simulink model "ON"  (R2025b)
settings: Solver=VariableStepAuto  StartTime=0.0  StopTime=165.5984  FixedStep=0.5  RelTol=1e-3
InitFcn:
  | createRefStates;
  | mdlWks = get_param(gcs,'ModelWorkspace');
  | a = getVariable(mdlWks,'a');
  | b = getVariable(mdlWks,'b');
  | c = getVariable(mdlWks,'c');
StopFcn:
  | fTraj = findobj("Tag","asbAUVTrajectory");
  | 
  | if isempty(fTraj)
  |    fTraj = figure("Tag","asbAUVTrajectory");
  |    axes(fTraj);
  | end
  | 
  | axTraj= gca(fTraj);
  | 
  | if exist('PositionData', 'var')
  |     % plot the intermediate points in yellow
  | 
  |    if d.Data == 1
  |       plot3(axTraj,ref_positions_x,ref_positions_y,ref_positions_z,'y*')
  |       hold on
  |       plot3(axTraj,PositionData(1,1),PositionData(1,2),PositionData(1,3),'r*')
  |       plot3(axTraj,PositionData(:,1),PositionData(:,2),PositionData(:,3));
  |       plot3(axTraj,PositionData(end,1),PositionData(end,2),PositionData(end,3),'g*');
  |       view(axTraj, 3);
  |    else
  |       plot(axTraj,ref_positions_x,ref_positions_y,'y*')
  |       hold on
  |       plot(axTraj,PositionData(1,1),PositionData(1,2),'r*')
  |       plot(axTraj,PositionData(:,1),PositionData(:,2));
  |       plot(axTraj,PositionData(end,1),PositionData(end,2),'g*');
  |       view(axTraj, 2);
  |    end
  | 
  | 
  | 
  | if exist("imu_acc", "var")
  | skip = 1;
  | N  = size(imu_acc.Data,1);
  | dt = (20/N)*skip;
  | T = N*dt;
  | 
  | % disp(["N", num2str(N)]);
  | % disp(["total time", num2str(T)]);
  | 
  | acc_bias = [0.0002;-0.00015;0.0001];
  | 
  | %% State vector
  | % x = [x y z vx vy vz bax bay baz]
  | n = 9;
  | 
  | %% True initial state
  | % x_true = [0;0;0;1;0.5;0.2];
  | 
  | %% Initial estimate
  | x_est = [PositionData(1,:)'; zeros(n-3,1)];
  | 
  | %% Initial covariance
  | P = 0.1*eye(n)*1;
  | 
  | %% Process noise
  | Q = diag([0 0 0 0.01 0.01 0.01 1e-6 1e-6 1e-6]);
  | % Q = diag([0 0 0 0.0 0.0 0.0 0 0 0]);
  | 
  | %% IMU noise
  | imu_noise = 0.02;
  | ... (+134 lines)
model workspace (MAT data in the model file):
  a = 0
  b = 1
  c = 1
  d = 0
values from neighbouring files (symbols this model uses):
  current_field = Config.water_current_params.field    [asbAUVax.m]
  data = [ ref_positions_x,           ref_positions_y,           ref_positions_z ]    [createRefStates.m]    (also in createRefStates_2D.m)
  imu_acc = acc_true + true_acc_bias + imu_noise*randn(3,1)    [covariance_examples.m]
  sampleTime = 0.1    [createRefStates.m]    (also in createRefStates_2D.m = 0.01)
  water_current_params = []    [createRefStates.m]
undefined symbols (not defined in the file or in its folder): obstacle_params
libraries: asbAUVlib x26, slpidlib x12, dspfdesign x6, aerolibobsolete x1, aerolibasang x1, sharedutil x1, aerolibnav x1, SignalEditorBlockLib x1
(part 3 of 3)

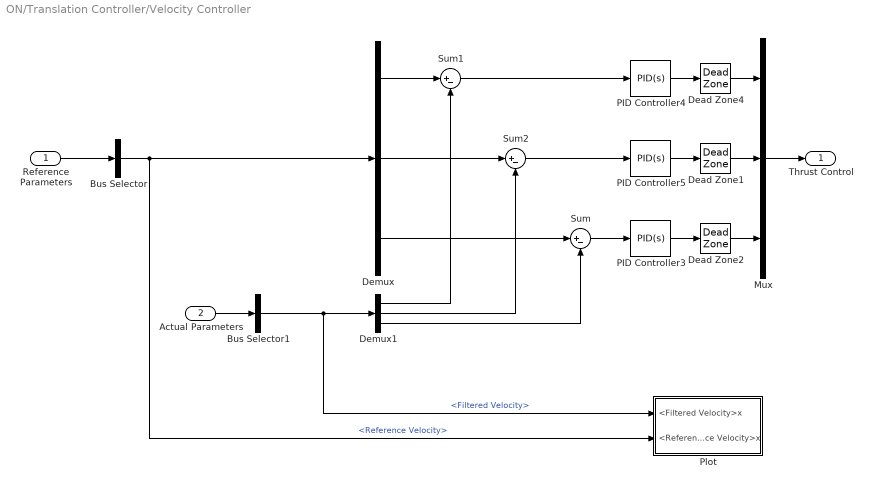
== system ON/Translation Controller/Velocity Controller ==
  Reference Parameters : Inport
  Actual Parameters : Inport  Port=2
  Bus Selector : BusSelector  OutputSignals=Reference Velocity
  Bus Selector1 : BusSelector  OutputSignals=Filtered Velocity
  Dead Zone1 : DeadZone  LowerValue=-0.05  UpperValue=+0.05
  Dead Zone2 : DeadZone  LowerValue=-0.05  UpperValue=+0.05
  Dead Zone4 : DeadZone  LowerValue=-0.05  UpperValue=+0.05
  Demux : Demux  Outputs=3
  Demux1 : Demux  Outputs=3
  Mux : Mux  Inputs=3
  PID Controller3 : slpidlib/PID Controller  Controller=PID  Form=Parallel  TimeDomain=Continuous-time  UseExternalTs=off  SampleTime=-1  IntegratorMethod=Forward Euler  FilterMethod=Forward Euler  ControllerParametersSource=internal  P=-0.61964554396314  I=-0.140214385843897  UseKiTs=off  D=0.00440045709674139  UseExternalDerivativeSource=off  N=140.813904178727  UseFilter=on  TunerSelectOption=Transfer Function Based (PID Tuner App)  InitialConditionSource=internal  InitialConditionForIntegrator=0  InitialConditionForFilter=0  DifferentiatorICPrevScaledInput=0  ExternalReset=none  TrackingMode=off  Kt=1  LimitOutput=off  SatLimitsSource=internal  UpperSaturationLimit=inf  LowerSaturationLimit=-inf  LinearizeAsGain=on  AntiWindupMode=none  Kb=1  LimitIntegrator=off  UpperIntegratorSaturationLimit=inf  LowerIntegratorSaturationLimit=-inf  POutMin=[]  POutMax=[]  IOutMin=[]  IOutMax=[]  DOutMin=[]  DOutMax=[]  NOutMin=[]  NOutMax=[]  SumOutMin=[]  SumOutMax=[]  SaturationOutMin=[]  SaturationOutMax=[]  PParamMin=[]  PParamMax=[]  IParamMin=[]  IParamMax=[]  DParamMin=[]  DParamMax=[]  NParamMin=[]  NParamMax=[]  KbParamMin=[]  KbParamMax=[]  KtParamMin=[]  KtParamMax=[]  KbOutMin=[]  KbOutMax=[]  KtOutMin=[]  KtOutMax=[]  IntegratorOutMin=[]  IntegratorOutMax=[]  FilterOutMin=[]  FilterOutMax=[]  SumI1OutMin=[]  SumI1OutMax=[]  SumI2OutMin=[]  SumI2OutMax=[]  SumI3OutMin=[]  SumI3OutMax=[]  SumI4OutMin=[]  SumI4OutMax=[]  SumDOutMin=[]  SumDOutMax=[]  DifferentiatorOutMin=[]  DifferentiatorOutMax=[]  FilterDiffOutCoefMin=[]  FilterDiffOutCoefMax=[]  ReciprocalOutMin=[]  ReciprocalOutMax=[]  SumDenOutMin=[]  SumDenOutMax=[]  SumNumOutMin=[]  SumNumOutMax=[]  DivideOutMin=[]  DivideOutMax=[]  UdiffTsProdOutMin=[]  UdiffTsProdOutMax=[]  NTsProdOutMin=[]  NTsProdOutMax=[]  UintegralTsProdOutMin=[]  UintegralTsProdOutMax=[]  UngainTsProdOutMin=[]  UngainTsProdOutMax=[]  ClampingZeroOutDataTypeStr=Inherit: Inherit via back propagation  ClampingZeroOutMin=[]  ClampingZeroOutMax=[]  FilterDenConstantOutDataTypeStr=Inherit: Inherit via back propagation  FilterDenConstantOutMin=[]  FilterDenConstantOutMax=[]  PCopyOutDataTypeStr=Inherit: Inherit via back propagation  PCopyOutMin=[]  PCopyOutMax=[]  NCopyOutDataTypeStr=Inherit: Inherit via back propagation  NCopyOutMin=[]  NCopyOutMax=[]  IntegratorContinuousStateAttributes=''  IntegratorStateMustResolveToSignalObject=off  IntegratorRTWStateStorageClass=Auto  FilterContinuousStateAttributes=''  FilterStateMustResolveToSignalObject=off  FilterRTWStateStorageClass=Auto  ParallelPVariant=InternalParameters  IdealPVariant=Disabled  IVariant=InternalParameters  DVariant=InternalParameters  IntegratorVariant=Continuous  SatVariant=Disabled  AWVariant=Passthrough  PCopyVariant=Disabled  TRVariant=Disabled  FdbkBlocksVariant=Forward  IdealPFdbkVariant=Disabled  SatFdbkVariant=Disabled  DerivativeFilterVariant=ContFilter  NVariant=InternalParameters  NCopyVariant=Disabled  FilterICVariant=InternalICsFilter  IntegratorICVariant=InternalICs  ExternalResetVariant=Disabled  TRSumVariant=Passthrough  SumFdbkVariant=Disabled  SumVariant=Sum_PID  TsampFilterVariant=InternalTs  TsampNgainVariant=Passthrough  TsampIntegralVariant=Disabled_SignalSpec  ExternalSaturationOutDataTypeStr=Inherit: Same as second input  DerivativeSourceVariant=ErrorSignal  PreIntVariant=InternalPreInt
  PID Controller4 : slpidlib/PID Controller  Controller=PID  Form=Parallel  TimeDomain=Continuous-time  UseExternalTs=off  SampleTime=-1  IntegratorMethod=Forward Euler  FilterMethod=Forward Euler  ControllerParametersSource=internal  P=0.262050505979025  I=0.0518732197045156  UseKiTs=off  D=-0.0235509594288088  UseExternalDerivativeSource=off  N=11.1269567072699  UseFilter=on  TunerSelectOption=Transfer Function Based (PID Tuner App)  InitialConditionSource=internal  InitialConditionForIntegrator=0  InitialConditionForFilter=0  DifferentiatorICPrevScaledInput=0  ExternalReset=none  TrackingMode=off  Kt=1  LimitOutput=off  SatLimitsSource=internal  UpperSaturationLimit=inf  LowerSaturationLimit=-inf  LinearizeAsGain=on  AntiWindupMode=none  Kb=1  LimitIntegrator=off  UpperIntegratorSaturationLimit=inf  LowerIntegratorSaturationLimit=-inf  POutMin=[]  POutMax=[]  IOutMin=[]  IOutMax=[]  DOutMin=[]  DOutMax=[]  NOutMin=[]  NOutMax=[]  SumOutMin=[]  SumOutMax=[]  SaturationOutMin=[]  SaturationOutMax=[]  PParamMin=[]  PParamMax=[]  IParamMin=[]  IParamMax=[]  DParamMin=[]  DParamMax=[]  NParamMin=[]  NParamMax=[]  KbParamMin=[]  KbParamMax=[]  KtParamMin=[]  KtParamMax=[]  KbOutMin=[]  KbOutMax=[]  KtOutMin=[]  KtOutMax=[]  IntegratorOutMin=[]  IntegratorOutMax=[]  FilterOutMin=[]  FilterOutMax=[]  SumI1OutMin=[]  SumI1OutMax=[]  SumI2OutMin=[]  SumI2OutMax=[]  SumI3OutMin=[]  SumI3OutMax=[]  SumI4OutMin=[]  SumI4OutMax=[]  SumDOutMin=[]  SumDOutMax=[]  DifferentiatorOutMin=[]  DifferentiatorOutMax=[]  FilterDiffOutCoefMin=[]  FilterDiffOutCoefMax=[]  ReciprocalOutMin=[]  ReciprocalOutMax=[]  SumDenOutMin=[]  SumDenOutMax=[]  SumNumOutMin=[]  SumNumOutMax=[]  DivideOutMin=[]  DivideOutMax=[]  UdiffTsProdOutMin=[]  UdiffTsProdOutMax=[]  NTsProdOutMin=[]  NTsProdOutMax=[]  UintegralTsProdOutMin=[]  UintegralTsProdOutMax=[]  UngainTsProdOutMin=[]  UngainTsProdOutMax=[]  ClampingZeroOutDataTypeStr=Inherit: Inherit via back propagation  ClampingZeroOutMin=[]  ClampingZeroOutMax=[]  FilterDenConstantOutDataTypeStr=Inherit: Inherit via back propagation  FilterDenConstantOutMin=[]  FilterDenConstantOutMax=[]  PCopyOutDataTypeStr=Inherit: Inherit via back propagation  PCopyOutMin=[]  PCopyOutMax=[]  NCopyOutDataTypeStr=Inherit: Inherit via back propagation  NCopyOutMin=[]  NCopyOutMax=[]  IntegratorContinuousStateAttributes=''  IntegratorStateMustResolveToSignalObject=off  IntegratorRTWStateStorageClass=Auto  FilterContinuousStateAttributes=''  FilterStateMustResolveToSignalObject=off  FilterRTWStateStorageClass=Auto  ParallelPVariant=InternalParameters  IdealPVariant=Disabled  IVariant=InternalParameters  DVariant=InternalParameters  IntegratorVariant=Continuous  SatVariant=Disabled  AWVariant=Passthrough  PCopyVariant=Disabled  TRVariant=Disabled  FdbkBlocksVariant=Forward  IdealPFdbkVariant=Disabled  SatFdbkVariant=Disabled  DerivativeFilterVariant=ContFilter  NVariant=InternalParameters  NCopyVariant=Disabled  FilterICVariant=InternalICsFilter  IntegratorICVariant=InternalICs  ExternalResetVariant=Disabled  TRSumVariant=Passthrough  SumFdbkVariant=Disabled  SumVariant=Sum_PID  TsampFilterVariant=InternalTs  TsampNgainVariant=Passthrough  TsampIntegralVariant=Disabled_SignalSpec  ExternalSaturationOutDataTypeStr=Inherit: Same as second input  DerivativeSourceVariant=ErrorSignal  PreIntVariant=InternalPreInt
  PID Controller5 : slpidlib/PID Controller  Controller=PID  Form=Parallel  TimeDomain=Continuous-time  UseExternalTs=off  SampleTime=-1  IntegratorMethod=Forward Euler  FilterMethod=Forward Euler  ControllerParametersSource=internal  P=1.14371295451496  I=0.548529610159355  UseKiTs=off  D=-0.00383210771245667  UseExternalDerivativeSource=off  N=298.455325458939  UseFilter=on  TunerSelectOption=Transfer Function Based (PID Tuner App)  InitialConditionSource=internal  InitialConditionForIntegrator=0  InitialConditionForFilter=0  DifferentiatorICPrevScaledInput=0  ExternalReset=none  TrackingMode=off  Kt=1  LimitOutput=off  SatLimitsSource=internal  UpperSaturationLimit=inf  LowerSaturationLimit=-inf  LinearizeAsGain=on  AntiWindupMode=none  Kb=1  LimitIntegrator=off  UpperIntegratorSaturationLimit=inf  LowerIntegratorSaturationLimit=-inf  POutMin=[]  POutMax=[]  IOutMin=[]  IOutMax=[]  DOutMin=[]  DOutMax=[]  NOutMin=[]  NOutMax=[]  SumOutMin=[]  SumOutMax=[]  SaturationOutMin=[]  SaturationOutMax=[]  PParamMin=[]  PParamMax=[]  IParamMin=[]  IParamMax=[]  DParamMin=[]  DParamMax=[]  NParamMin=[]  NParamMax=[]  KbParamMin=[]  KbParamMax=[]  KtParamMin=[]  KtParamMax=[]  KbOutMin=[]  KbOutMax=[]  KtOutMin=[]  KtOutMax=[]  IntegratorOutMin=[]  IntegratorOutMax=[]  FilterOutMin=[]  FilterOutMax=[]  SumI1OutMin=[]  SumI1OutMax=[]  SumI2OutMin=[]  SumI2OutMax=[]  SumI3OutMin=[]  SumI3OutMax=[]  SumI4OutMin=[]  SumI4OutMax=[]  SumDOutMin=[]  SumDOutMax=[]  DifferentiatorOutMin=[]  DifferentiatorOutMax=[]  FilterDiffOutCoefMin=[]  FilterDiffOutCoefMax=[]  ReciprocalOutMin=[]  ReciprocalOutMax=[]  SumDenOutMin=[]  SumDenOutMax=[]  SumNumOutMin=[]  SumNumOutMax=[]  DivideOutMin=[]  DivideOutMax=[]  UdiffTsProdOutMin=[]  UdiffTsProdOutMax=[]  NTsProdOutMin=[]  NTsProdOutMax=[]  UintegralTsProdOutMin=[]  UintegralTsProdOutMax=[]  UngainTsProdOutMin=[]  UngainTsProdOutMax=[]  ClampingZeroOutDataTypeStr=Inherit: Inherit via back propagation  ClampingZeroOutMin=[]  ClampingZeroOutMax=[]  FilterDenConstantOutDataTypeStr=Inherit: Inherit via back propagation  FilterDenConstantOutMin=[]  FilterDenConstantOutMax=[]  PCopyOutDataTypeStr=Inherit: Inherit via back propagation  PCopyOutMin=[]  PCopyOutMax=[]  NCopyOutDataTypeStr=Inherit: Inherit via back propagation  NCopyOutMin=[]  NCopyOutMax=[]  IntegratorContinuousStateAttributes=''  IntegratorStateMustResolveToSignalObject=off  IntegratorRTWStateStorageClass=Auto  FilterContinuousStateAttributes=''  FilterStateMustResolveToSignalObject=off  FilterRTWStateStorageClass=Auto  ParallelPVariant=InternalParameters  IdealPVariant=Disabled  IVariant=InternalParameters  DVariant=InternalParameters  IntegratorVariant=Continuous  SatVariant=Disabled  AWVariant=Passthrough  PCopyVariant=Disabled  TRVariant=Disabled  FdbkBlocksVariant=Forward  IdealPFdbkVariant=Disabled  SatFdbkVariant=Disabled  DerivativeFilterVariant=ContFilter  NVariant=InternalParameters  NCopyVariant=Disabled  FilterICVariant=InternalICsFilter  IntegratorICVariant=InternalICs  ExternalResetVariant=Disabled  TRSumVariant=Passthrough  SumFdbkVariant=Disabled  SumVariant=Sum_PID  TsampFilterVariant=InternalTs  TsampNgainVariant=Passthrough  TsampIntegralVariant=Disabled_SignalSpec  ExternalSaturationOutDataTypeStr=Inherit: Same as second input  DerivativeSourceVariant=ErrorSignal  PreIntVariant=InternalPreInt
  Plot : Subsystem  AncestorBlock=asbAUVlib/Plot
  Sum : Sum  Inputs=|+-
  Sum1 : Sum  Inputs=|+-
  Sum2 : Sum  Inputs=|+-
  Thrust Control : Outport  VectorParamsAs1DForOutWhenUnconnected=off
  wires:
  Demux1/3 -> Sum/2
  PID Controller3/1 -> Dead Zone2/1
  Demux/3 -> Sum/1
  PID Controller4/1 -> Dead Zone4/1
  PID Controller5/1 -> Dead Zone1/1
  Demux/2 -> Sum2/1
  Dead Zone2/1 -> Mux/3
  Dead Zone1/1 -> Mux/2
  Demux/1 -> Sum1/1
  Demux1/1 -> Sum1/2
  Demux1/2 -> Sum2/2
  Dead Zone4/1 -> Mux/1
  Mux/1 -> Thrust Control/1
  Sum1/1 -> PID Controller4/1
  Sum2/1 -> PID Controller5/1
  Sum/1 -> PID Controller3/1
  Bus Selector/1 -> Plot/2(<Reference Velocity>x), Demux/1  "<Reference Velocity>"
  Reference Parameters/1 -> Bus Selector/1
  Bus Selector1/1 -> Plot/1(<Filtered Velocity>x), Demux1/1  "<Filtered Velocity>"
  Actual Parameters/1 -> Bus Selector1/1

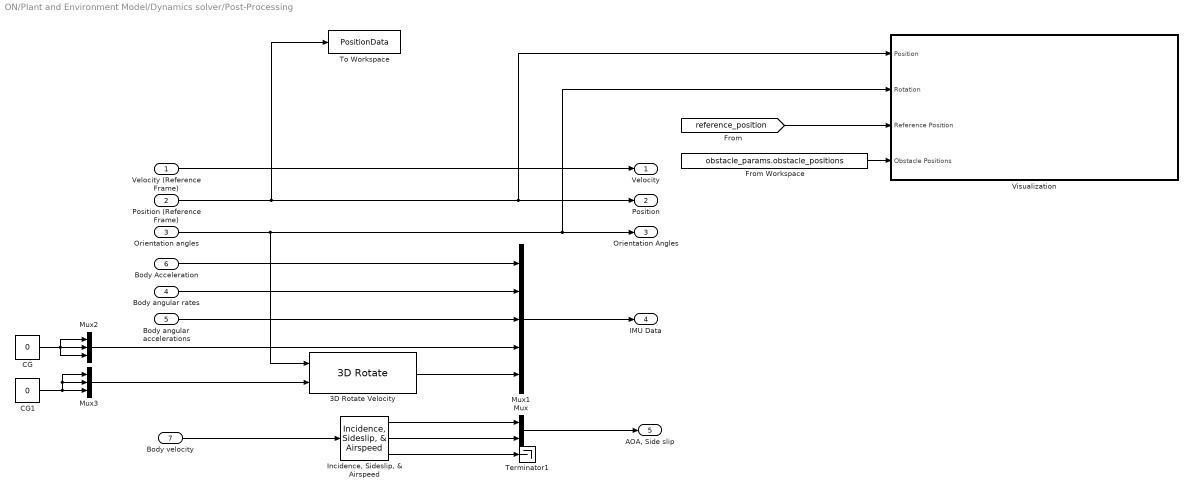
== system ON/Plant and Environment Model/Dynamics solver/Post-Processing ==
  Velocity (Reference Frame) : Inport
  Position (Reference Frame) : Inport  Port=2
  Orientation angles : Inport  Port=3
  Body angular rates : Inport  Port=4
  Body angular accelerations : Inport  Port=5
  Body Acceleration : Inport  Port=6
  Body velocity : Inport  Port=7
  3D Rotate Velocity : asbAUVlib/3D Rotate   SystemSampleTime=-1  VariantActivationTime=update diagram  EmptyChoice=off  PassThrough=off  PassThroughVariantControl=(default)  EmptyChoiceVariantControl=(default)  AllowFlexibleInterface=on  Latency=0  AutoFrameSizeCalculation=off
  CG : Constant  Value=0
  CG1 : Constant  Value=0
  From Workspace : FromWorkspace  VariableName=obstacle_params.obstacle_positions
  "Incidence, Sideslip, & Airspeed" : aerolibasang/Incidence, Sideslip, & Airspeed
  Mux : Mux  Inputs=2
  Mux1 : Mux  Inputs=5
  Mux2 : Mux  Inputs=3
  Mux3 : Mux  Inputs=3
  Terminator1 : Terminator
  To Workspace : ToWorkspace  VariableName=PositionData  SampleTime=-1
  Visualization : Subsystem  mask(6DoF_Animation){u2=sampleTime*10, u8=on, u9=d, u10=water_current_params, u11=obstacle_params}
      mask prompts: u2 "aeroblks:aeroblkanim6dof:block6DoF_AnimationParamTimeintervalbetweenupdates"; u8 "aeroblks:aeroblkanim6dof:block6DoF_AnimationParamEnableanimation"; u9 "2D or 3D plotting"; u10 "Water Current Parameters"; u11 "Obstacle Parameters"
      mask help: aeroblks:aeroblkanim6dof:block6DoF_AnimationDesc
      mask init:
      | aeroicon('aeroblk');
      | Config.update = u2;
      | Config.Animenable = u8;
      | Config.Model = bdroot(gcb);
      | Config.dimension = u9;
      | Config.water_current_params = u10;
      | Config.obstacle_params = u11;
      mask Help: eval('asbhelp(''sixdof_animation'')');
      mask DialogControl DescGroupVar Prompt: Animation
      mask DialogControl DescTextVar Prompt: Show animation of body
      mask DialogControl u2 Prompt: Time interval between updates:
      mask DialogControl u8 Prompt: Enable animation
      mask Display:
      | port_label('input',1,'x_e','texmode','on');
      | port_label('input',2,'\phi \theta \psi','texmode','on');
  Velocity : Outport  VectorParamsAs1DForOutWhenUnconnected=off
  " Position" : Outport  Port=2  VectorParamsAs1DForOutWhenUnconnected=off
  Orientation Angles : Outport  Port=3  VectorParamsAs1DForOutWhenUnconnected=off
  IMU Data : Outport  Port=4  VectorParamsAs1DForOutWhenUnconnected=off
  "AOA, Side slip" : Outport  Port=5  VectorParamsAs1DForOutWhenUnconnected=off
  wires:
  Body angular accelerations/1 -> Mux1/3
  "Incidence, Sideslip, & Airspeed"/2 -> Mux/2
  Body velocity/1 -> "Incidence, Sideslip, & Airspeed"/1
  "Incidence, Sideslip, & Airspeed"/1 -> Mux/1
  Body angular rates/1 -> Mux1/2
  CG/1 -> Mux2/2, Mux2/1, Mux2/3
  3D Rotate Velocity/1 -> Mux1/5
  Mux2/1 -> Mux1/4
  Mux/1 -> "AOA, Side slip"/1
  CG1/1 -> Mux3/2, Mux3/1, Mux3/3
  Mux3/1 -> 3D Rotate Velocity/2
  Body Acceleration/1 -> Mux1/1
  Velocity (Reference Frame)/1 -> Velocity/1
  Orientation angles/1 -> 3D Rotate Velocity/1, Visualization/2(Rotation), Orientation Angles/1
  Mux1/1 -> IMU Data/1
  "Incidence, Sideslip, & Airspeed"/3 -> Terminator1/1
  Position (Reference Frame)/1 -> " Position"/1, Visualization/1(Position), To Workspace/1
  [reference_position] -> Visualization/3(Reference Position)
  From Workspace/1 -> Visualization/4(Obstacle Positions)

== system ON/Plant and Environment Model/Environmental Forces & Moments/Hydrodynamic Forces ==
  "Submarine Velocity (Body Axis) " : Inport
  "AOA, Side Slip" : Inport  Port=2
  Hydrodynamic Forces - Accurate : Subsystem  VariantControl=b==1
  Hydrodynamic Forces - Basic : Subsystem  VariantControl=b==0
  "Force due to Lift, Drag" : Outport  VectorParamsAs1DForOutWhenUnconnected=off

== system ON/Plant and Environment Model/Environmental Forces & Moments/Hydrostatic Forces ==
  In1 : Inport
  Constant : Constant
  Environment Model : Subsystem  mask{ro=1000, V=0.01, M=10, a=0, b=0, c=0}
      mask prompts: ro "Density of Water"; V "Volume of Submarine"; M "Mass of Submarine"; a "X Distance between CG and CB"; b "Y Distance between CG and CB"; c "Z Distance between CG and CB"
      mask DialogControl DescTextVar Prompt: Enter the Submarine related Parameters
      mask DialogControl Container3 Prompt: Distance between CG and Center of Buoyancy
  Hydrostatic Force : Outport  VectorParamsAs1DForOutWhenUnconnected=off
  Hydrostatic Moment : Outport  Port=2  VectorParamsAs1DForOutWhenUnconnected=off
  wires:
  Constant/1 -> Environment Model/1("Fraction submerged ")
  Environment Model/2(Moment due to Weight and Buoyancy) -> Hydrostatic Moment/1
  Environment Model/1(Forces due to Weight and Buoyancy) -> Hydrostatic Force/1
  In1/1 -> Environment Model/2(Orientation Angles)

== system ON/Plant and Environment Model/Propulsion Forces & Moments/Force and moments due to Thrust ==
  Thrust Inputs : Inport
  "Thrust to Propulsion " : Subsystem
  Propulsion Force : Outport  VectorParamsAs1DForOutWhenUnconnected=off
  Propulsion Moment : Outport  Port=2  VectorParamsAs1DForOutWhenUnconnected=off
  wires:
  "Thrust to Propulsion "/2(Propulsion Moment) -> Propulsion Moment/1
  Thrust Inputs/1 -> "Thrust to Propulsion "/1(Thrust Inputs)
  "Thrust to Propulsion "/1(Propulsion Force) -> Propulsion Force/1

== system ON/Plant and Environment Model/Propulsion Forces & Moments/Input commands to Thrust ==
  Thrust Control Inputs : Inport
  Demux : Demux  Outputs=3
  Input Commands to PWM : Subsystem
  "PWM Signals to Thrust " : Subsystem
  Thrust values : Outport  VectorParamsAs1DForOutWhenUnconnected=off
  wires:
  Input Commands to PWM/1(Px1) -> "PWM Signals to Thrust "/1(PWM Signal Px1)
  Input Commands to PWM/3(Py1) -> "PWM Signals to Thrust "/3(PWM Signal Py1)
  Demux/1 -> Input Commands to PWM/1(X Thruster)  "X Thrust Input"
  Demux/3 -> Input Commands to PWM/3(Z Thruster)  "Z Thrust Input"
  Input Commands to PWM/4(Py2) -> "PWM Signals to Thrust "/4(PWM Signal Py2)
  Demux/2 -> Input Commands to PWM/2(Y Thruster)  "Y Thrust Input"
  Input Commands to PWM/2(Px2) -> "PWM Signals to Thrust "/2(PWM Signal Px2)
  Input Commands to PWM/5(Pz) -> "PWM Signals to Thrust "/5(PWM Signal Pz)
  "PWM Signals to Thrust "/1(Thrust (N)) -> Thrust values/1
  Thrust Control Inputs/1 -> Demux/1

== system ON/Sensor data and State Estimation/System With Noise/ Sensor (IMU) ==
  IMU Inputs : Inport
  Bus Creator : BusCreator  Inputs=2
  Bus Selector : BusSelector  OutputSignals=IMU Data
  Demux : Demux  Outputs=5
  Three-axis Inertial Measurement Unit : aerolibnav/Three-axis Inertial Measurement Unit  units=Metric (MKS)  imu=data(1,:)  i_Ts=0  dtype_a=on  w_a=190  z_a=0.707  a_sf_cc=[1 0 0; 0 1 0; 0 0 1]  a_bias=[0 0 0]  a_sat="[-inf  -inf  -inf  inf inf inf]"  dtype_g=on  w_g=190  z_g=0.707  g_sf_cc=[1 0 0; 0 1 0; 0 0 1]  g_bias=[0 0 0]  g_sens=[0 0 0]  g_sat="[-inf  -inf  -inf  inf inf inf]"  i_rand=on  i_seeds=[23093 23094 23095 23096 23097 23098]  i_pow=[0.00001 0.00001 0.00001 0.00001 0.00001 0.00001]
  IMU Measurements : Outport  VectorParamsAs1DForOutWhenUnconnected=off
  wires:
  Three-axis Inertial Measurement Unit/1 -> Bus Creator/1  "IMU Measured Acceleration"
  Demux/2 -> Three-axis Inertial Measurement Unit/2
  Demux/4 -> Three-axis Inertial Measurement Unit/4
  Demux/5 -> Three-axis Inertial Measurement Unit/5
  Demux/3 -> Three-axis Inertial Measurement Unit/3
  Demux/1 -> Three-axis Inertial Measurement Unit/1
  Three-axis Inertial Measurement Unit/2 -> Bus Creator/2  "IMU Measured Body Rates"
  IMU Inputs/1 -> Bus Selector/1
  Bus Selector/1 -> Demux/1  "<IMU Data>"
  Bus Creator/1 -> IMU Measurements/1

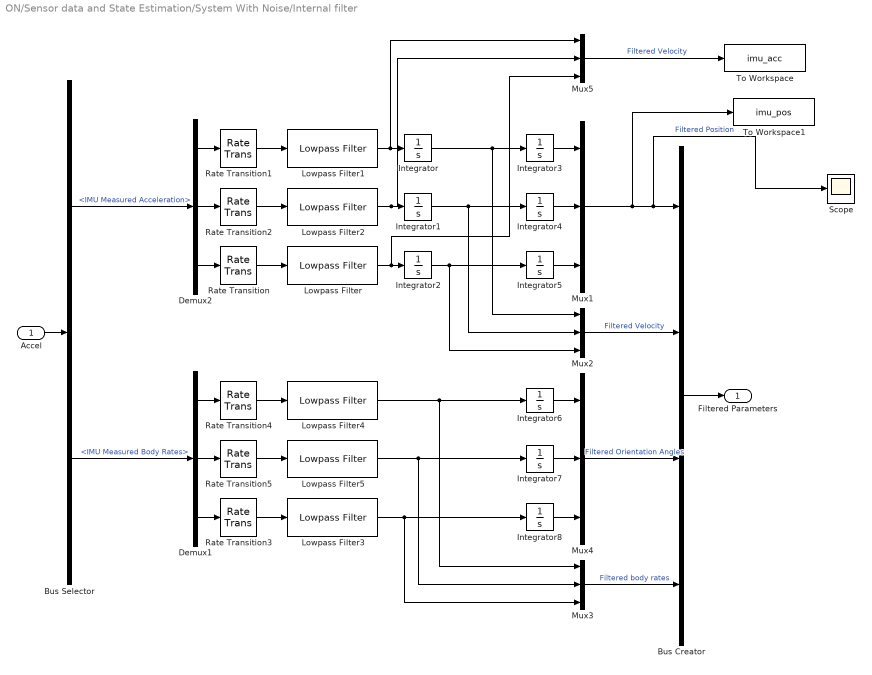
== system ON/Sensor data and State Estimation/System With Noise/Internal filter ==
  Accel : Inport
  Bus Creator : BusCreator  Inputs=4
  Bus Selector : BusSelector  OutputSignals=IMU Measured Acceleration,IMU Measured Body Rates
  Demux1 : Demux  Outputs=3
  Demux2 : Demux  Outputs=3
  Integrator{,1..2,6..8} (6 alike) : Integrator
  Integrator3 : Integrator  InitialCondition=data(1,1)
  Integrator4 : Integrator  InitialCondition=data(1,2)
  Integrator5 : Integrator  InitialCondition=data(1,3)
  Lowpass Filter{,1..5} (6 alike) : dspfdesign/Lowpass Filter  FilterType=FIR  DesignForMinimumOrder=on  FilterOrder=50  PassbandFrequency=1/100  StopbandFrequency=45  PassbandRipple=0.1  StopbandAttenuation=80  SampleRateMode=Specify on dialog  SampleRate=100  SimulateUsing=Interpreted execution  roundingMode=Floor  coeffsDataTypeStr=fixdt(1,16)
  Mux{1..5} (5 alike) : Mux  Inputs=3
  Rate Transition{,1..5} (6 alike) : RateTransition  OutPortSampleTime=0.01
  Scope : Scope
      settings: ActiveDisplayYMinimum=-560.24422155517175  ActiveDisplayYMaximum=62.268150319716625
  To Workspace : ToWorkspace  VariableName=imu_acc  SaveFormat=Timeseries  SampleTime=-1
  To Workspace1 : ToWorkspace  VariableName=imu_pos  SaveFormat=Timeseries  SampleTime=-1
  Filtered Parameters : Outport  VectorParamsAs1DForOutWhenUnconnected=off
  wires:
  Rate Transition5/1 -> Lowpass Filter5/1
  Rate Transition4/1 -> Lowpass Filter4/1
  Demux1/1 -> Rate Transition4/1
  Lowpass Filter3/1 -> Integrator8/1, Mux3/3
  Demux1/2 -> Rate Transition5/1
  Lowpass Filter5/1 -> Integrator7/1, Mux3/2
  Lowpass Filter4/1 -> Integrator6/1, Mux3/1
  Integrator6/1 -> Mux4/1
  Rate Transition3/1 -> Lowpass Filter3/1
  Integrator8/1 -> Mux4/3
  Demux1/3 -> Rate Transition3/1
  Integrator7/1 -> Mux4/2
  Accel/1 -> Bus Selector/1
  Bus Selector/1 -> Demux2/1  "<IMU Measured Acceleration>"
  Bus Selector/2 -> Demux1/1  "<IMU Measured Body Rates>"
  Mux4/1 -> Bus Creator/3  "Filtered Orientation Angles"
  Mux3/1 -> Bus Creator/4  "Filtered body rates"
  Bus Creator/1 -> Filtered Parameters/1
  Integrator2/1 -> Integrator5/1, Mux2/3
  Integrator/1 -> Integrator3/1, Mux2/1
  Mux2/1 -> Bus Creator/2  "Filtered Velocity"
  Mux1/1 -> To Workspace1/1, Scope/1, Bus Creator/1  "Filtered Position"
  Lowpass Filter/1 -> Mux5/3, Integrator2/1
  Demux2/2 -> Rate Transition2/1
  Rate Transition1/1 -> Lowpass Filter1/1
  Integrator4/1 -> Mux1/2
  Demux2/3 -> Rate Transition/1
  Lowpass Filter2/1 -> Mux5/2, Integrator1/1
  Lowpass Filter1/1 -> Mux5/1, Integrator/1
  Demux2/1 -> Rate Transition1/1
  Integrator5/1 -> Mux1/3
  Integrator1/1 -> Integrator4/1, Mux2/2
  Rate Transition/1 -> Lowpass Filter/1
  Integrator3/1 -> Mux1/1
  Rate Transition2/1 -> Lowpass Filter2/1
  Mux5/1 -> To Workspace/1  "Filtered Velocity"

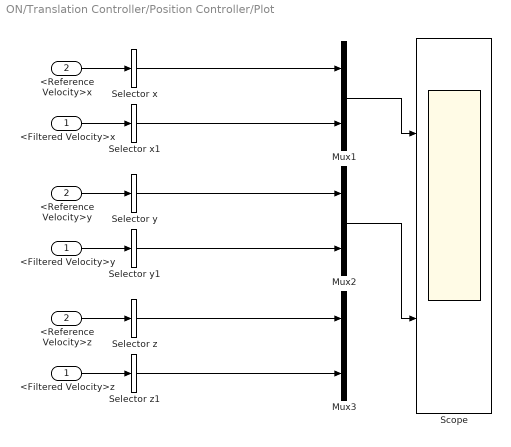
== system ON/Translation Controller/Position Controller/Plot ==
  <Filtered Velocity>x : Inport
  <Reference Velocity>x : Inport  Port=2
  <Filtered Velocity>y : InportShadow
  <Filtered Velocity>z : InportShadow
  <Reference Velocity>y : InportShadow  Port=2
  <Reference Velocity>z : InportShadow  Port=2
  Mux1 : Mux  Inputs=2
  Mux2 : Mux  Inputs=2
  Mux3 : Mux  Inputs=2
  Scope : Scope  NumInputPorts=2
      settings: ActiveDisplayYMinimum=-3.1120995154510725E+7  ActiveDisplayYMaximum=3.4601198502526991E+6
  Selector x : Selector  InputPortWidth=3  IndexOptions=Index vector (dialog)  Indices=1  OutputSizes=1
  Selector x1 : Selector  InputPortWidth=3  IndexOptions=Index vector (dialog)  Indices=1  OutputSizes=1
  Selector y : Selector  InputPortWidth=3  IndexOptions=Index vector (dialog)  Indices=2  OutputSizes=1
  Selector y1 : Selector  InputPortWidth=3  IndexOptions=Index vector (dialog)  Indices=2  OutputSizes=1
  Selector z : Selector  InputPortWidth=3  IndexOptions=Index vector (dialog)  Indices=2  OutputSizes=1
  Selector z1 : Selector  InputPortWidth=3  IndexOptions=Index vector (dialog)  Indices=2  OutputSizes=1
  wires:
  <Filtered Velocity>z/1 -> Selector z1/1
  <Filtered Velocity>y/1 -> Selector y1/1
  <Filtered Velocity>x/1 -> Selector x1/1
  <Reference Velocity>z/1 -> Selector z/1
  <Reference Velocity>y/1 -> Selector y/1
  <Reference Velocity>x/1 -> Selector x/1
  Selector z1/1 -> Mux3/2
  Selector x/1 -> Mux1/1
  Selector y/1 -> Mux2/1
  Mux1/1 -> Scope/1
  Mux2/1 -> Scope/2
  Selector z/1 -> Mux3/1
  Selector y1/1 -> Mux2/2
  Selector x1/1 -> Mux1/2

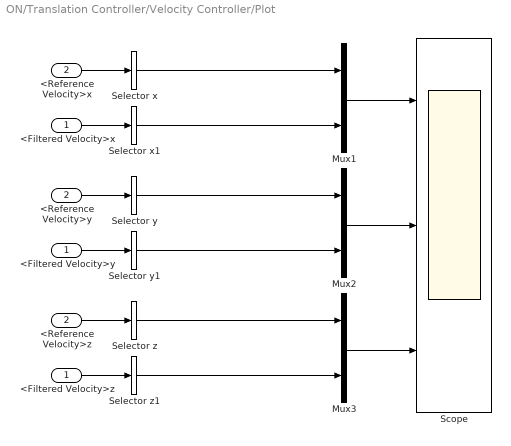
== system ON/Translation Controller/Velocity Controller/Plot ==
  <Filtered Velocity>x : Inport
  <Reference Velocity>x : Inport  Port=2
  <Filtered Velocity>y : InportShadow
  <Filtered Velocity>z : InportShadow
  <Reference Velocity>y : InportShadow  Port=2
  <Reference Velocity>z : InportShadow  Port=2
  Mux1 : Mux  Inputs=2
  Mux2 : Mux  Inputs=2
  Mux3 : Mux  Inputs=2
  Scope : Scope  NumInputPorts=3
      settings: ActiveDisplayYMinimum=-1  ActiveDisplayYMaximum=1
  Selector x : Selector  InputPortWidth=3  IndexOptions=Index vector (dialog)  Indices=1  OutputSizes=1
  Selector x1 : Selector  InputPortWidth=3  IndexOptions=Index vector (dialog)  Indices=1  OutputSizes=1
  Selector y : Selector  InputPortWidth=3  IndexOptions=Index vector (dialog)  Indices=2  OutputSizes=1
  Selector y1 : Selector  InputPortWidth=3  IndexOptions=Index vector (dialog)  Indices=2  OutputSizes=1
  Selector z : Selector  InputPortWidth=3  IndexOptions=Index vector (dialog)  Indices=2  OutputSizes=1
  Selector z1 : Selector  InputPortWidth=3  IndexOptions=Index vector (dialog)  Indices=2  OutputSizes=1
  wires:
  <Filtered Velocity>z/1 -> Selector z1/1
  <Filtered Velocity>y/1 -> Selector y1/1
  <Filtered Velocity>x/1 -> Selector x1/1
  <Reference Velocity>z/1 -> Selector z/1
  <Reference Velocity>y/1 -> Selector y/1
  <Reference Velocity>x/1 -> Selector x/1
  Selector z1/1 -> Mux3/2
  Selector x/1 -> Mux1/1
  Selector y/1 -> Mux2/1
  Mux1/1 -> Scope/1
  Mux2/1 -> Scope/2
  Selector z/1 -> Mux3/1
  Selector y1/1 -> Mux2/2
  Selector x1/1 -> Mux1/2
  Mux3/1 -> Scope/3

== system ON/Plant and Environment Model/Dynamics solver/Post-Processing/Visualization ==
  Position : Inport
  Rotation : Inport  Port=2  Unit=rad
  Reference Position : Inport  Port=3
  Obstacle Positions : Inport  Port=4
  Animation S-Function : M-S-Function  FunctionName=asbAUVax  Parameters=Config
  Mux4 : Mux  Inputs=2
  wires:
  Rotation/1 -> Mux4/2
  Mux4/1 -> Animation S-Function/1
  Position/1 -> Mux4/1
  Reference Position/1 -> Animation S-Function/2
  Obstacle Positions/1 -> Animation S-Function/3

== system ON/Plant and Environment Model/Environmental Forces & Moments/Hydrodynamic Forces/Hydrodynamic Forces - Accurate ==
  note: Source of Equations:
      | Submarine Dynamic Modeling, by
      | Dr Peter Ridley Julien Fontan and Dr Peter Corke
      |
      | Part: Hydrodynamic forces and moments
  "Submarine Velocity (Body Axis) " : Inport
  "AOA, Side Slip" : Inport  Port=2
  "AOA, Side Slip1" : InportShadow  Port=2
  Marine Drag - Body axes : asbAUVlib/Marine Drag - Body - Accurate  SystemSampleTime=-1  VariantActivationTime=update diagram  EmptyChoice=off  PassThrough=off  PassThroughVariantControl=(default)  EmptyChoiceVariantControl=(default)  AllowFlexibleInterface=on  Latency=0  AutoFrameSizeCalculation=off
  Marine Lift - Body axes : asbAUVlib/Marine Lift - Body - Accurate  SystemSampleTime=-1  VariantActivationTime=update diagram  EmptyChoice=off  PassThrough=off  PassThroughVariantControl=(default)  EmptyChoiceVariantControl=(default)  AllowFlexibleInterface=on  Latency=0  AutoFrameSizeCalculation=off
  Submarine Velocity (Body Axis) 1 : InportShadow
  Sum : Sum
  "Force due to Lift, Drag" : Outport  VectorParamsAs1DForOutWhenUnconnected=off
  wires:
  Marine Drag - Body axes/1 -> Sum/1
  Marine Lift - Body axes/1 -> Sum/2
  "AOA, Side Slip"/1 -> Marine Drag - Body axes/2
  "Submarine Velocity (Body Axis) "/1 -> Marine Drag - Body axes/1
  Sum/1 -> "Force due to Lift, Drag"/1
  "AOA, Side Slip1"/1 -> Marine Lift - Body axes/2
  Submarine Velocity (Body Axis) 1/1 -> Marine Lift - Body axes/1

== system ON/Plant and Environment Model/Environmental Forces & Moments/Hydrodynamic Forces/Hydrodynamic Forces - Basic ==
  "Submarine Velocity (Body Axis) " : Inport
  "AOA, Side Slip" : Inport  Port=2
  "AOA, Side Slip1" : InportShadow  Port=2
  Marine Drag - Body Axes : Subsystem  AncestorBlock=asbAUVlib/Marine Drag - Body - Approximate
  Marine Lift - Body Axes : asbAUVlib/Marine Lift - Body - Approximate  SystemSampleTime=-1  VariantActivationTime=update diagram  EmptyChoice=off  PassThrough=off  PassThroughVariantControl=(default)  EmptyChoiceVariantControl=(default)  AllowFlexibleInterface=on  Latency=0  AutoFrameSizeCalculation=off
  Submarine Velocity (Body Axis) 1 : InportShadow
  Sum : Sum
  "Force due to Lift, Drag" : Outport  VectorParamsAs1DForOutWhenUnconnected=off
  wires:
  Marine Drag - Body Axes/1(Drag Forces in Body Axis) -> Sum/1
  Marine Lift - Body Axes/1 -> Sum/2
  "AOA, Side Slip"/1 -> Marine Lift - Body Axes/2
  "Submarine Velocity (Body Axis) "/1 -> Marine Drag - Body Axes/1(Marine Velocities in Body Axis)
  Sum/1 -> "Force due to Lift, Drag"/1
  "AOA, Side Slip1"/1 -> Marine Drag - Body Axes/2(AOA and Side Slip)
  Submarine Velocity (Body Axis) 1/1 -> Marine Lift - Body Axes/1

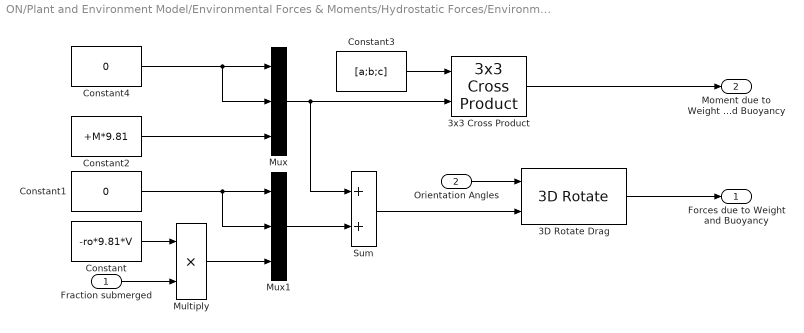
== system ON/Plant and Environment Model/Environmental Forces & Moments/Hydrostatic Forces/Environment Model ==
  "Fraction submerged " : Inport
  Orientation Angles : Inport  Port=2
  3D Rotate Drag : asbAUVlib/3D Rotate   SystemSampleTime=-1  VariantActivationTime=update diagram  EmptyChoice=off  PassThrough=off  PassThroughVariantControl=(default)  EmptyChoiceVariantControl=(default)  AllowFlexibleInterface=on  Latency=0  AutoFrameSizeCalculation=off
  3x3 Cross Product : sharedutil/3x3 Cross Product  aMode=aMode
      settings: LibrarySourceBlock=aerolibutil/3x3 Cross Product
  Constant : Constant  Value=-ro*9.81*V
  Constant1 : Constant  Value=0
  Constant2 : Constant  Value=+M*9.81
  Constant3 : Constant  Value=[a;b;c]
  Constant4 : Constant  Value=0
  Multiply : Product
  Mux : Mux  Inputs=3
  Mux1 : Mux  Inputs=3
  Sum : Sum
  Forces due to Weight and Buoyancy : Outport  VectorParamsAs1DForOutWhenUnconnected=off
  Moment due to Weight and Buoyancy : Outport  Port=2  VectorParamsAs1DForOutWhenUnconnected=off
  wires:
  3x3 Cross Product/1 -> Moment due to Weight and Buoyancy/1
  Constant3/1 -> 3x3 Cross Product/1
  "Fraction submerged "/1 -> Multiply/2
  Mux1/1 -> Sum/2
  Multiply/1 -> Mux1/3
  Mux/1 -> 3x3 Cross Product/2, Sum/1
  Constant/1 -> Multiply/1
  Constant1/1 -> Mux1/2, Mux1/1
  Constant2/1 -> Mux/3
  Sum/1 -> 3D Rotate Drag/2
  Orientation Angles/1 -> 3D Rotate Drag/1
  3D Rotate Drag/1 -> Forces due to Weight and Buoyancy/1
  Constant4/1 -> Mux/1, Mux/2

== system ON/Plant and Environment Model/Propulsion Forces & Moments/Force and moments due to Thrust/Thrust to Propulsion  ==
  Thrust Inputs : Inport
  Demux : Demux  Outputs=5
  Moment computation : Subsystem
  Sum : Sum  Inputs=+++++
  Thrust Transformation : Subsystem
  Propulsion Force : Outport  VectorParamsAs1DForOutWhenUnconnected=off
  Propulsion Moment : Outport  Port=2  VectorParamsAs1DForOutWhenUnconnected=off
  wires:
  Demux/5 -> Moment computation/5(Pz)
  Demux/4 -> Moment computation/4(Py2)
  Demux/3 -> Moment computation/3(Py1)
  Demux/2 -> Moment computation/2(Px2)
  Demux/1 -> Moment computation/1(Px1)
  Thrust Transformation/3(Thrust Py1) -> Sum/3
  Moment computation/1(Moment) -> Propulsion Moment/1
  Thrust Transformation/4(Thrust Py2) -> Sum/4
  Thrust Transformation/5(Thrust Pz) -> Sum/5
  Sum/1 -> Propulsion Force/1
  Thrust Inputs/1 -> Thrust Transformation/1(Thrust Inputs), Demux/1
  Thrust Transformation/1(Thrust Px1) -> Sum/1
  Thrust Transformation/2(Thrust Px2) -> Sum/2

== system ON/Plant and Environment Model/Propulsion Forces & Moments/Input commands to Thrust/Input Commands to PWM ==
  X Thruster : Inport
  Y Thruster : Inport  Port=2
  Z Thruster : Inport  Port=3
  Control2PWM X : asbAUVlib/Control2PWM Subsystem  SystemSampleTime=-1  VariantActivationTime=update diagram  EmptyChoice=off  PassThrough=off  PassThroughVariantControl=(default)  EmptyChoiceVariantControl=(default)  AllowFlexibleInterface=on  Latency=0  AutoFrameSizeCalculation=off
  Control2PWM Y : asbAUVlib/Control2PWM Subsystem  SystemSampleTime=-1  VariantActivationTime=update diagram  EmptyChoice=off  PassThrough=off  PassThroughVariantControl=(default)  EmptyChoiceVariantControl=(default)  AllowFlexibleInterface=on  Latency=0  AutoFrameSizeCalculation=off
  Control2PWM Z : asbAUVlib/Control2PWM Subsystem  SystemSampleTime=-1  VariantActivationTime=update diagram  EmptyChoice=off  PassThrough=off  PassThroughVariantControl=(default)  EmptyChoiceVariantControl=(default)  AllowFlexibleInterface=on  Latency=0  AutoFrameSizeCalculation=off
  Px1 : Outport  VectorParamsAs1DForOutWhenUnconnected=off
  Px2 : Outport  Port=2  VectorParamsAs1DForOutWhenUnconnected=off
  Py1 : Outport  Port=3  VectorParamsAs1DForOutWhenUnconnected=off
  Py2 : Outport  Port=4  VectorParamsAs1DForOutWhenUnconnected=off
  Pz : Outport  Port=5  VectorParamsAs1DForOutWhenUnconnected=off
  wires:
  Control2PWM Z/1 -> Pz/1
  Y Thruster/1 -> Control2PWM Y/1
  Control2PWM Y/1 -> Py1/1, Py2/1
  Z Thruster/1 -> Control2PWM Z/1
  Control2PWM X/1 -> Px1/1, Px2/1
  X Thruster/1 -> Control2PWM X/1

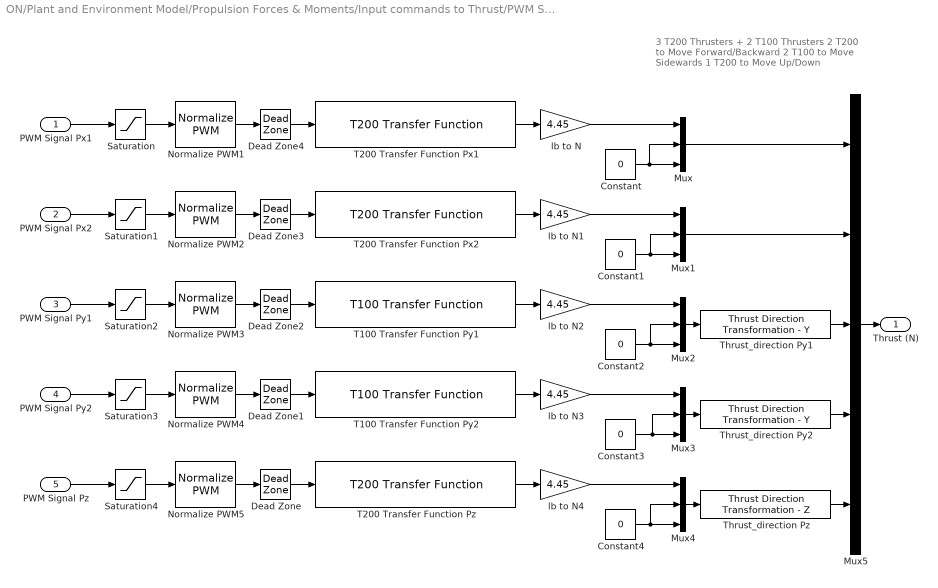
== system ON/Plant and Environment Model/Propulsion Forces & Moments/Input commands to Thrust/PWM Signals to Thrust  ==
  note: 3 T200 Thrusters + 2 T100 Thrusters
      |
      | 2 T200 to Move Forward/Backward
      | 2 T100 to Move Sidewards
      | 1 T200 to Move Up/Down
  PWM Signal Px1 : Inport
  PWM Signal Px2 : Inport  Port=2
  PWM Signal Py1 : Inport  Port=3
  PWM Signal Py2 : Inport  Port=4
  PWM Signal Pz : Inport  Port=5
  Constant{,1..4} (5 alike) : Constant  Value=0
  Dead Zone{,2..4} (4 alike) : DeadZone  LowerValue=-10  UpperValue=+10
  Dead Zone1 : DeadZone  LowerValue=-10  UpperValue=10
  Mux{,1..4} (5 alike) : Mux  Inputs=3
  Mux5 : Mux  Inputs=5
  Normalize PWM{1..5} (5 alike) : asbAUVlib/Normalize PWM  SystemSampleTime=-1  VariantActivationTime=update diagram  EmptyChoice=off  PassThrough=off  PassThroughVariantControl=(default)  EmptyChoiceVariantControl=(default)  AllowFlexibleInterface=on  Latency=0  AutoFrameSizeCalculation=off
  Saturation{,1..4} (5 alike) : Saturate  UpperLimit=1900  LowerLimit=1100
  T100 Transfer Function Py1 : asbAUVlib/T100 Transfer Function  SystemSampleTime=-1  VariantActivationTime=update diagram  EmptyChoice=off  PassThrough=off  PassThroughVariantControl=(default)  EmptyChoiceVariantControl=(default)  AllowFlexibleInterface=on  Latency=0  AutoFrameSizeCalculation=off
  T100 Transfer Function Py2 : asbAUVlib/T100 Transfer Function  SystemSampleTime=-1  VariantActivationTime=update diagram  EmptyChoice=off  PassThrough=off  PassThroughVariantControl=(default)  EmptyChoiceVariantControl=(default)  AllowFlexibleInterface=on  Latency=0  AutoFrameSizeCalculation=off
  T200 Transfer Function Px1 : asbAUVlib/T200 Transfer Function  SystemSampleTime=-1  VariantActivationTime=update diagram  EmptyChoice=off  PassThrough=off  PassThroughVariantControl=(default)  EmptyChoiceVariantControl=(default)  AllowFlexibleInterface=on  Latency=0  AutoFrameSizeCalculation=off
  T200 Transfer Function Px2 : asbAUVlib/T200 Transfer Function  SystemSampleTime=-1  VariantActivationTime=update diagram  EmptyChoice=off  PassThrough=off  PassThroughVariantControl=(default)  EmptyChoiceVariantControl=(default)  AllowFlexibleInterface=on  Latency=0  AutoFrameSizeCalculation=off
  T200 Transfer Function Pz : asbAUVlib/T200 Transfer Function  SystemSampleTime=-1  VariantActivationTime=update diagram  EmptyChoice=off  PassThrough=off  PassThroughVariantControl=(default)  EmptyChoiceVariantControl=(default)  AllowFlexibleInterface=on  Latency=0  AutoFrameSizeCalculation=off
  Thrust_direction Py1 : asbAUVlib/Thrust Direction Transformation - Y  SystemSampleTime=-1  VariantActivationTime=update diagram  EmptyChoice=off  PassThrough=off  PassThroughVariantControl=(default)  EmptyChoiceVariantControl=(default)  AllowFlexibleInterface=on  Latency=0  AutoFrameSizeCalculation=off
  Thrust_direction Py2 : asbAUVlib/Thrust Direction Transformation - Y  SystemSampleTime=-1  VariantActivationTime=update diagram  EmptyChoice=off  PassThrough=off  PassThroughVariantControl=(default)  EmptyChoiceVariantControl=(default)  AllowFlexibleInterface=on  Latency=0  AutoFrameSizeCalculation=off
  Thrust_direction Pz : asbAUVlib/Thrust Direction Transformation - Z  SystemSampleTime=-1  VariantActivationTime=update diagram  EmptyChoice=off  PassThrough=off  PassThroughVariantControl=(default)  EmptyChoiceVariantControl=(default)  AllowFlexibleInterface=on  Latency=0  AutoFrameSizeCalculation=off
  lb to N{,1..4} (5 alike) : Gain  Gain=4.45
  Thrust (N) : Outport  VectorParamsAs1DForOutWhenUnconnected=off
  wires:
  Dead Zone3/1 -> T200 Transfer Function Px2/1
  Dead Zone1/1 -> T100 Transfer Function Py2/1
  Dead Zone/1 -> T200 Transfer Function Pz/1
  Normalize PWM5/1 -> Dead Zone/1
  Normalize PWM4/1 -> Dead Zone1/1
  Normalize PWM3/1 -> Dead Zone2/1
  Normalize PWM2/1 -> Dead Zone3/1
  Saturation3/1 -> Normalize PWM4/1
  PWM Signal Py2/1 -> Saturation3/1
  Saturation4/1 -> Normalize PWM5/1
  Saturation2/1 -> Normalize PWM3/1
  Saturation1/1 -> Normalize PWM2/1
  Saturation/1 -> Normalize PWM1/1
  Normalize PWM1/1 -> Dead Zone4/1
  T100 Transfer Function Py2/1 -> lb to N3/1
  lb to N2/1 -> Mux2/1
  Mux4/1 -> Thrust_direction Pz/1
  Mux5/1 -> Thrust (N)/1
  Thrust_direction Pz/1 -> Mux5/5
  lb to N/1 -> Mux/1
  Constant1/1 -> Mux1/2, Mux1/3
  T200 Transfer Function Px2/1 -> lb to N1/1
  Mux3/1 -> Thrust_direction Py2/1
  PWM Signal Pz/1 -> Saturation4/1
  PWM Signal Px1/1 -> Saturation/1
  Constant/1 -> Mux/2, Mux/3
  Thrust_direction Py2/1 -> Mux5/4
  Thrust_direction Py1/1 -> Mux5/3
  PWM Signal Py1/1 -> Saturation2/1
  Mux1/1 -> Mux5/2
  lb to N1/1 -> Mux1/1
  lb to N4/1 -> Mux4/1
  Constant4/1 -> Mux4/3, Mux4/2
  T200 Transfer Function Pz/1 -> lb to N4/1
  Mux/1 -> Mux5/1
  Constant2/1 -> Mux2/3, Mux2/2
  Mux2/1 -> Thrust_direction Py1/1
  PWM Signal Px2/1 -> Saturation1/1
  Constant3/1 -> Mux3/2, Mux3/3
  lb to N3/1 -> Mux3/1
  Dead Zone4/1 -> T200 Transfer Function Px1/1
  T200 Transfer Function Px1/1 -> lb to N/1
  Dead Zone2/1 -> T100 Transfer Function Py1/1
  T100 Transfer Function Py1/1 -> lb to N2/1

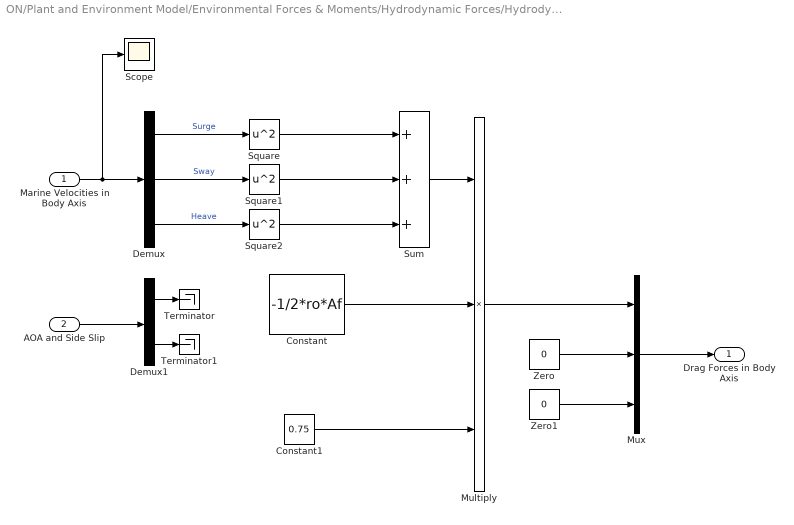
== system ON/Plant and Environment Model/Environmental Forces & Moments/Hydrodynamic Forces/Hydrodynamic Forces - Basic/Marine Drag - Body Axes ==
  Marine Velocities in Body Axis : Inport
  AOA and Side Slip : Inport  Port=2
  Constant : Constant  Value=-1/2*ro*Af  mask{ro=1000, Af=0.001}
      mask prompts: ro "Density of Water"; Af "Submarine Frontal Area"
      mask DialogControl DescGroupVar Prompt: Input
      mask DialogControl DescTextVar Prompt: Enter the following values :
  Constant1 : Constant  Value=0.75
  Demux : Demux  Outputs=3
  Demux1 : Demux  Outputs=2
  Multiply : Product  Inputs=3
  Mux : Mux  Inputs=3
  Scope : Scope
      settings: ActiveDisplayYMinimum=-19.523269050125279  ActiveDisplayYMaximum=15.815981669268936  DataLoggingVariableName=ScopeData5
  Square : Math  Operator=square  SignedPower=on
  Square1 : Math  Operator=square  SignedPower=on
  Square2 : Math  Operator=square  SignedPower=on
  Sum : Sum  Inputs=+++
  Terminator : Terminator
  Terminator1 : Terminator
  Zero : Constant  Value=0  OutDataTypeStr=Inherit: Inherit via back propagation
  Zero1 : Constant  Value=0  OutDataTypeStr=Inherit: Inherit via back propagation
  Drag Forces in Body Axis : Outport  VectorParamsAs1DForOutWhenUnconnected=off
  wires:
  Zero1/1 -> Mux/3
  Zero/1 -> Mux/2
  Multiply/1 -> Mux/1
  Constant1/1 -> Multiply/3
  Constant/1 -> Multiply/2
  Demux1/2 -> Terminator1/1
  Demux1/1 -> Terminator/1
  Square1/1 -> Sum/2
  Square/1 -> Sum/1
  Demux/2 -> Square1/1  "Sway"
  Demux/1 -> Square/1  "Surge"
  Sum/1 -> Multiply/1
  Demux/3 -> Square2/1  "Heave"
  Square2/1 -> Sum/3
  Mux/1 -> Drag Forces in Body Axis/1
  Marine Velocities in Body Axis/1 -> Scope/1, Demux/1
  AOA and Side Slip/1 -> Demux1/1

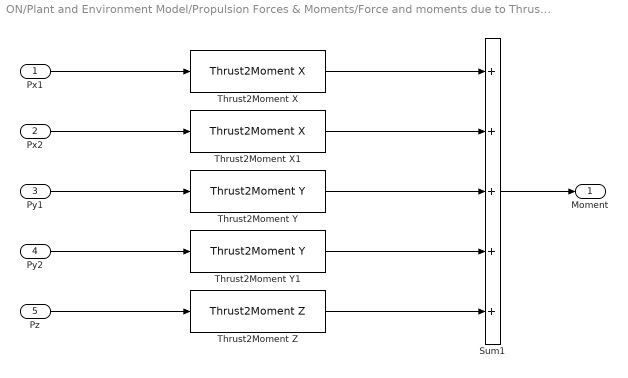
== system ON/Plant and Environment Model/Propulsion Forces & Moments/Force and moments due to Thrust/Thrust to Propulsion /Moment computation ==
  Px1 : Inport
  Px2 : Inport  Port=2
  Py1 : Inport  Port=3
  Py2 : Inport  Port=4
  Pz : Inport  Port=5
  Sum1 : Sum  Inputs=+++++
  Thrust2Moment X : asbAUVlib/Thrust2Moment X  a=0  b=-0.2  c=0
  Thrust2Moment X1 : asbAUVlib/Thrust2Moment X  a=0  b=0.2  c=0
  Thrust2Moment Y : asbAUVlib/Thrust2Moment Y  a=.2  b=0  c=0
  Thrust2Moment Y1 : asbAUVlib/Thrust2Moment Y  a=-0.2  b=0  c=0
  Thrust2Moment Z : asbAUVlib/Thrust2Moment Z  a=0  b=0  c=0
  Moment : Outport  VectorParamsAs1DForOutWhenUnconnected=off
  wires:
  Py2/1 -> Thrust2Moment Y1/1
  Px1/1 -> Thrust2Moment X/1
  Py1/1 -> Thrust2Moment Y/1
  Thrust2Moment X/1 -> Sum1/1
  Thrust2Moment X1/1 -> Sum1/2
  Thrust2Moment Z/1 -> Sum1/5
  Thrust2Moment Y1/1 -> Sum1/4
  Pz/1 -> Thrust2Moment Z/1
  Thrust2Moment Y/1 -> Sum1/3
  Sum1/1 -> Moment/1
  Px2/1 -> Thrust2Moment X1/1

== system ON/Plant and Environment Model/Propulsion Forces & Moments/Force and moments due to Thrust/Thrust to Propulsion /Thrust Transformation ==
  Thrust Inputs : Inport
  Demux1 : Demux  Outputs=5
  Thrust Px1 : Outport  VectorParamsAs1DForOutWhenUnconnected=off
  Thrust Px2 : Outport  Port=2  VectorParamsAs1DForOutWhenUnconnected=off
  Thrust Py1 : Outport  Port=3  VectorParamsAs1DForOutWhenUnconnected=off
  Thrust Py2 : Outport  Port=4  VectorParamsAs1DForOutWhenUnconnected=off
  Thrust Pz : Outport  Port=5  VectorParamsAs1DForOutWhenUnconnected=off
  wires:
  Demux1/4 -> Thrust Py2/1
  Demux1/5 -> Thrust Pz/1
  Thrust Inputs/1 -> Demux1/1
  Demux1/1 -> Thrust Px1/1
  Demux1/2 -> Thrust Px2/1
  Demux1/3 -> Thrust Py1/1

== matlab function ON/Plant and Environment Model/Environmental Forces & Moments/MATLAB Function ==
  data: actual_position input; F_rep output; obstacle_positions input; d_3D input
function F_rep = potential_field(actual_position, obstacle_positions, d_3D)
k_rep = 20000000;
d0 = 100.0;  % kilometers

F_rep = [0;0;0];

% for each obstacle
for i = 1:(size(obstacle_positions,1)/3)
    obs = obstacle_positions((1:3)+(i-1)*3,1);
    dist = norm(actual_position - obs);
    % disp(obs)
    % disp(d)
    if dist < d0
        unit_vector = (actual_position - obs) / dist;
        F_rep = k_rep * (1/dist - 1/d0) * (1/(dist^2)) * unit_vector;
        % F_rep = k_rep * (obs - actual_position);
        % disp(F_rep);
        if ~d_3D
            F_rep(3) = 0;
        end
        % disp(F_rep);
    end

end
